simulink model "P4_ObsvSmlk"  (R2015a)
settings: Solver=ode45  StartTime=0.0  StopTime=15  FixedStep=1e-6  RelTol=1e-3
values from neighbouring files (symbols this model uses):
  A = [-1 -3 0;0 1 1; 0 2 0]    [P2_MinRealz.m]
  B = [ 1 2/3; 0 1/3; 0 1/3]    [P2_MinRealz.m]
  C = [1 -1 2;0  6 3]    [P2_MinRealz.m]
  D = [0 -1/3; 0 0]    [P2_MinRealz.m]
undefined symbols (not defined in the file or in its folder): Aobs, Bobs, Cobs, Dobs, K, x0, x0obs
settings Model: Creator=paiva  LastModifiedBy=paiva
settings SolverCC: ShapePreserveControl=EnableAll

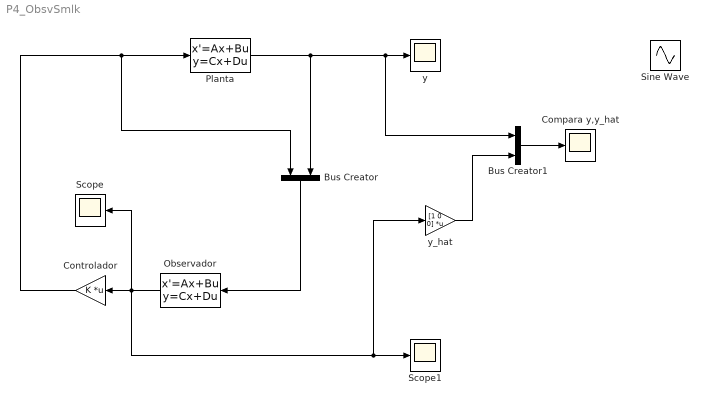
== system P4_ObsvSmlk ==
  Bus Creator : BusCreator  Inputs=2
  Bus Creator1 : BusCreator  Inputs=2
  Compara y,y_hat : Scope
      settings: SaveName=ScopeData3
  Controlador : Gain  Gain=K  Multiplication=Matrix(K*u) (u vector)
  Observador : StateSpace  A=Aobs  B=Bobs  C=Cobs  D=Dobs  X0=x0obs
  Planta : StateSpace  A=A  B=B  C=C  D=D  X0=x0
  Scope : Scope
  Scope1 : Scope
  Sine Wave : Sin  SampleTime=0
  y : Scope
      settings: SaveName=ScopeData2
  y_hat : Gain  Gain="[1  0 0]"  Multiplication=Matrix(K*u) (u vector)
  wires:
  Planta/1 -> Bus Creator1/1, y/1, Bus Creator/2
  Observador/1 -> y_hat/1, Scope1/1, Scope/1, Controlador/1
  Bus Creator/1 -> Observador/1
  Controlador/1 -> Bus Creator/1, Planta/1
  y_hat/1 -> Bus Creator1/2
  Bus Creator1/1 -> Compara y,y_hat/1
